simulink model "grading_system"  (R2018b)
settings: Solver=VariableStepAuto  StartTime=0.0  StopTime=10.0  RelTol=1e-3
settings Model: Creator=Conan  LastModifiedBy=Conan

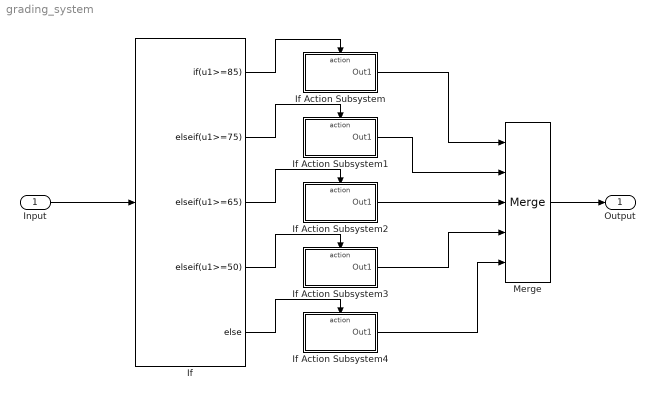
== system grading_system ==
  Input : Inport
  If : If  IfExpression=u1>=85  ElseIfExpressions=u1>=75,u1>=65,u1>=50
  If Action Subsystem : Subsystem  TreatAsAtomicUnit=on
  If Action Subsystem1 : Subsystem  TreatAsAtomicUnit=on
  If Action Subsystem2 : Subsystem  TreatAsAtomicUnit=on
  If Action Subsystem3 : Subsystem  TreatAsAtomicUnit=on
  If Action Subsystem4 : Subsystem  TreatAsAtomicUnit=on
  Merge : Merge  Inputs=5
  Output : Outport
  wires:
  If/1 -> If Action Subsystem/Action
  If/2 -> If Action Subsystem1/Action
  If/3 -> If Action Subsystem2/Action
  If/4 -> If Action Subsystem3/Action
  If/5 -> If Action Subsystem4/Action
  If Action Subsystem/1(Out1) -> Merge/1
  If Action Subsystem1/1(Out1) -> Merge/2
  If Action Subsystem2/1(Out1) -> Merge/3
  If Action Subsystem3/1(Out1) -> Merge/4
  If Action Subsystem4/1(Out1) -> Merge/5
  Merge/1 -> Output/1
  Input/1 -> If/1

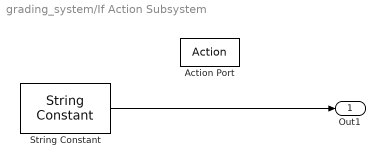
== system grading_system/If Action Subsystem ==
  Action Port : ActionPort  ActionType=then
  String Constant : StringConstant  String="\"Excelent\""
  Out1 : Outport
  wires:
  String Constant/1 -> Out1/1

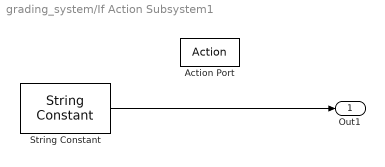
== system grading_system/If Action Subsystem1 ==
  Action Port : ActionPort  ActionType=elseif
  String Constant : StringConstant  String="\"Ver Good\""
  Out1 : Outport
  wires:
  String Constant/1 -> Out1/1

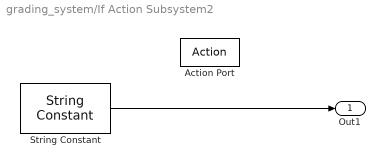
== system grading_system/If Action Subsystem2 ==
  Action Port : ActionPort  ActionType=elseif
  String Constant : StringConstant  String="\"Good\""
  Out1 : Outport
  wires:
  String Constant/1 -> Out1/1

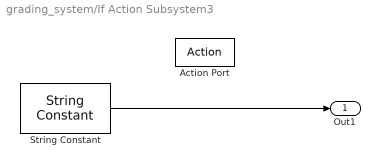
== system grading_system/If Action Subsystem3 ==
  Action Port : ActionPort  ActionType=elseif
  String Constant : StringConstant  String="\"Pass\""
  Out1 : Outport
  wires:
  String Constant/1 -> Out1/1

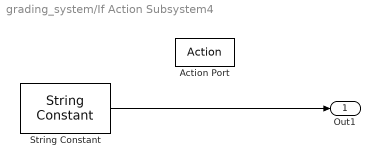
== system grading_system/If Action Subsystem4 ==
  Action Port : ActionPort  ActionType=else
  String Constant : StringConstant  String="\"Failed\""
  Out1 : Outport
  wires:
  String Constant/1 -> Out1/1
